simulink library "downlink_4c2t_lib"  (Simulink 8.7)
settings: Solver=ode45  StartTime=0.0  StopTime=10.0  RelTol=1e-3
PreLoadFcn:
  | LutContent = LUTS.ENTRIES;
InitFcn:
  | LutContent = LUTS.ENTRIES;
values from neighbouring files (symbols this model uses):
  cordic_gain = 1.8    [setup_downlink_4c2t.m]
undefined symbols (not defined in the file or in its folder): AdvDSPBDMemDisplay, dpoly, evalAionMaskParam, LUTS, UseDontCare, value
libraries: DSPBAPrim x42, DSPBAModelBus x10, DSPBAVectorUtil x2, downlink_4c2t_cordic_lib x1
settings Model: Creator=VMAUER  LastModifiedBy=5g

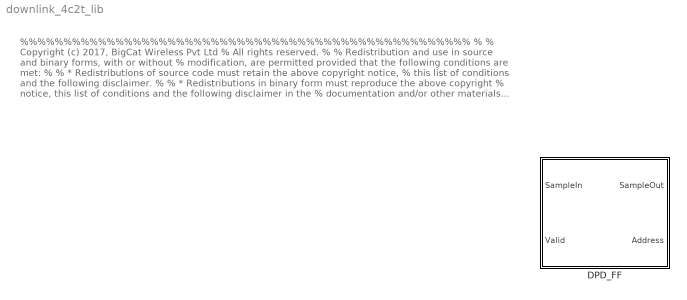
== system downlink_4c2t_lib ==
  note: %%%%%%%%%%%%%%%%%%%%%%%%%%%%%%%%%%%%%%%%%%%%%%%%%%%%
      |  %
      |  % Copyright (c) 2017, BigCat Wireless Pvt Ltd
      |  % All rights reserved.
      |  %
      |  % Redistribution and use in source and binary forms, with or without
      |  % modification, are permitted provided that the following conditions are met:
      |  %
      |  %     * Redistributions of source code must retain the above copyright notice,
      |  %       this list of conditions and the following disclaimer.
      |  %
      |  %     * Redistributions in binary form must reproduce the above copyright
      |  %       notice, this list of conditions and the following disclaimer in the
      |  %       documentation and/or other materials provided with the distribution.
      |  %
      |  %     * Neither the name of the copyright holder nor the names of its contributors
      |  %       may be used to endorse or promote products derived from this software
      |  %       without specific prior written permission.
      |  %
      |  %
      |  %
      |  % THIS SOFTWARE IS PROVIDED BY THE COPYRIGHT HOLDERS AND CONTRIBUTORS "AS IS"
      |  % AND ANY EXPRESS OR IMPLIED WARRANTIES, INCLUDING, BUT NOT LIMITED TO, THE
      |  % IMPLIED WARRANTIES OF MERCHANTABILITY AND FITNESS FOR A PARTICULAR PURPOSE ARE
      |  % DISCLAIMED. IN NO EVENT SHALL THE COPYRIGHT HOLDER OR CONTRIBUTORS BE LIABLE
      |  % FOR ANY DIRECT, INDIRECT, INCIDENTAL, SPECIAL, EXEMPLARY, OR CONSEQUENTIAL
      |  % DAMAGES (INCLUDING, BUT NOT LIMITED TO, PROCUREMENT OF SUBSTITUTE GOODS OR
      |  % SERVICES; LOSS OF USE, DATA, OR PROFITS; OR BUSINESS INTERRUPTION) HOWEVER
      |  % CAUSED AND ON ANY THEORY OF LIABILITY, WHETHER IN CONTRACT, STRICT LIABILITY,
      |  % OR TORT (INCLUDING NEGLIGENCE OR OTHERWISE) ARISING IN ANY WAY OUT OF THE USE
      |  % OF THIS SOFTWARE, EVEN IF ADVISED OF THE POSSIBILITY OF SUCH DAMAGE.
      |  %
      |   %%%%%%%%%%%%%%%%%%%%%%%%%%%%%%%%%%%%%%%%%%%%%%%%%%%%%
  DPD_FF : Subsystem  mask{LutContent=LUTS.ENTRIES, CoefWidth=16, Coeff_fractionwidth=11, DataWidth=16, fractionwidth=15, LutUpdateAddress=512, LutUpdateCoeff1=513, LutUpdateCoeff2=514, LutUpdateCoeff3=515, LutUpdateCoeff4=516, LutUpdateCoeff5=517, LutUpdateCoeff6=518, LutUpdateCoeff7=519, LutUpdateCoeff8=520, DPDReadBankAddress=521}
      mask prompts: LutContent "initial LUT content"; CoefWidth "Coefficient Width"; DataWidth "Data Width"; LutUpdateAddress "DPD LUT update address"; LutUpdateCoeff1 "DPD LUT update coeff 1"; LutUpdateCoeff2 "DPD LUT update coeff 2"; LutUpdateCoeff3 "DPD LUT update coeff 3"; LutUpdateCoeff4 "DPD LUT update coeff 4"; LutUpdateCoeff5 "DPD LUT update coeff 5"; LutUpdateCoeff6 "DPD LUT update coeff 6"; LutUpdateCoeff7 "DPD LUT update coeff 7"; LutUpdateCoeff8 "DPD LUT update coeff 8"; DPDReadBankAddress "DPD LUT read bank select"

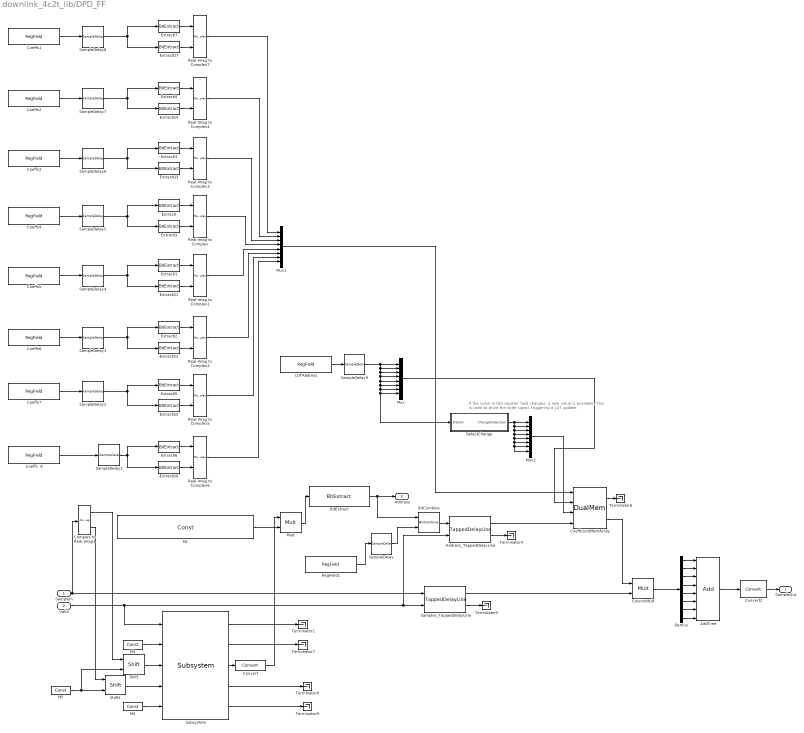
== system downlink_4c2t_lib/DPD_FF ==
  note: If the value in this register field changes, a new value is available.
      | This is used to drive the write signal, triggering a LUT update.
  SampleIn : Inport
  Valid : Inport  Port=2
  AddTree : DSPBAPrim/Add  primtype=add  nInputs=evalAionMaskParam(gcb,'value',1)  nOutputs=1  omode=Inherit via internal rule with word growth  otype=sfix(16)  scale=2^-15  rndmethod=Unbiased  factor=1  satmethod=Symmetric  shift_vec=[0 1 2 -1]  value=8  inPortNames=[' '; ' ';]  outPortNames=[' ']  dspbaimage=dspba_prim.jpg  text=fprintf('+');  style=Optimised  visibilities=1032+2^17+2^18+2^19  genFPC=off  floatRounding=correct  advOptions=[]  version=20130821
  Address_TappedDelayLine : DSPBAVectorUtil/TappedDelayLine  numTaps=size(LutContent, 2)  zeroOrOne=0  reverse=off
  BitCombine : DSPBAPrim/BitCombine  primtype=bitcombine  nInputs=2  nOutputs=1  omode=Inherit via internal rule  otype=sfix(16)  scale=2^-15  rndmethod=Unbiased  factor=1  satmethod=Symmetric  shift_vec=[0 1 2 -1]  value=0  inPortNames=['l'; 'h';]  outPortNames=[' ']  dspbaimage=dspba_prim.jpg  text=fprintf('[h,l]');  style=Optimised  visibilities=8+2  version=20090407
  BitExtract : DSPBAPrim/BitExtract  primtype=bitextract  nInputs=1  nOutputs=1  omode=Specify via dialog  otype=ufix(8)  scale=1  rndmethod=Unbiased  factor=1  satmethod=Symmetric  shift_vec=[0 1 2 -1]  value=log2(size(LutContent,1))  inPortNames=[' '; ' ';]  outPortNames=[' ']  dspbaimage=dspba_prim.jpg  text=fprintf('..%d', value);  style=Optimised  visibilities=8 + 1024  version=20090407
  CoefficientMemArray : DSPBAPrim/DualMem  primtype=dualmem  nInputs=4  nOutputs=2  omode=Specify via dialog  otype=sfix(CoefWidth)  scale=2^-Coeff_fractionwidth  rndmethod=Unbiased  factor=1  satmethod=Symmetric  shift_vec=[0 1 2 -1]  value=[LUTS.ENTRIES' LUTS.ENTRIES']'  inPortNames=['d'; 'a'; 'w'; 'a']  outPortNames=['q1'; 'q2']  dspbaimage=dspba_prim.jpg  text=fprintf('dmem%s',AdvDSPBDMemDisplay(UseDontCare));  style=Optimised  visibilities=8 + 1024 + 2^17  UseDontCare=on  TwinWritePorts=off  version=20141001
  Coeffs  8 : DSPBAModelBus/RegField  reg_name=LutUpdateCoeff8  reg_rwmode=Read/Write  reg_msb=2*DataWidth-1  reg_lsb=0  reg_mode=Specify via dialog  reg_type=ufix(2*DataWidth)  reg_scale=1  reg_init=0  reg_desc=I and Q coeffs for the next LUT entrance  reg_modal=off  reg_desc0=0  reg_desc1=0  reg_desc2=0  reg_desc3=0  reg_desc4=0  reg_desc5=0  reg_desc6=0  reg_desc7=0  reg_addr=520  SampleTime=-1  version=20090407
  Coeffs1 : DSPBAModelBus/RegField  reg_name=LutUpdateCoeff1  reg_rwmode=Read/Write  reg_msb=2*DataWidth-1  reg_lsb=0  reg_mode=Specify via dialog  reg_type=ufix(2*DataWidth)  reg_scale=1  reg_init=0  reg_desc=I and Q coeffs for the next LUT entrance  reg_modal=off  reg_desc0=0  reg_desc1=0  reg_desc2=0  reg_desc3=0  reg_desc4=0  reg_desc5=0  reg_desc6=0  reg_desc7=0  reg_addr=513  SampleTime=-1  version=20090407
  Coeffs2 : DSPBAModelBus/RegField  reg_name=LutUpdateCoeff2  reg_rwmode=Read/Write  reg_msb=2*DataWidth-1  reg_lsb=0  reg_mode=Specify via dialog  reg_type=ufix(2*DataWidth)  reg_scale=1  reg_init=0  reg_desc=I and Q coeffs for the next LUT entrance  reg_modal=off  reg_desc0=0  reg_desc1=0  reg_desc2=0  reg_desc3=0  reg_desc4=0  reg_desc5=0  reg_desc6=0  reg_desc7=0  reg_addr=514  SampleTime=-1  version=20090407
  Coeffs3 : DSPBAModelBus/RegField  reg_name=LutUpdateCoeff3  reg_rwmode=Read/Write  reg_msb=2*DataWidth-1  reg_lsb=0  reg_mode=Specify via dialog  reg_type=ufix(2*DataWidth)  reg_scale=1  reg_init=0  reg_desc=I and Q coeffs for the next LUT entrance  reg_modal=off  reg_desc0=0  reg_desc1=0  reg_desc2=0  reg_desc3=0  reg_desc4=0  reg_desc5=0  reg_desc6=0  reg_desc7=0  reg_addr=515  SampleTime=-1  version=20090407
  Coeffs4 : DSPBAModelBus/RegField  reg_name=LutUpdateCoeff4  reg_rwmode=Read/Write  reg_msb=2*DataWidth-1  reg_lsb=0  reg_mode=Specify via dialog  reg_type=ufix(2*DataWidth)  reg_scale=1  reg_init=0  reg_desc=I and Q coeffs for the next LUT entrance  reg_modal=off  reg_desc0=0  reg_desc1=0  reg_desc2=0  reg_desc3=0  reg_desc4=0  reg_desc5=0  reg_desc6=0  reg_desc7=0  reg_addr=516  SampleTime=-1  version=20090407
  Coeffs5 : DSPBAModelBus/RegField  reg_name=LutUpdateCoeff5  reg_rwmode=Read/Write  reg_msb=2*DataWidth-1  reg_lsb=0  reg_mode=Specify via dialog  reg_type=ufix(2*DataWidth)  reg_scale=1  reg_init=0  reg_desc=I and Q coeffs for the next LUT entrance  reg_modal=off  reg_desc0=0  reg_desc1=0  reg_desc2=0  reg_desc3=0  reg_desc4=0  reg_desc5=0  reg_desc6=0  reg_desc7=0  reg_addr=517  SampleTime=-1  version=20090407
  Coeffs6 : DSPBAModelBus/RegField  reg_name=LutUpdateCoeff6  reg_rwmode=Read/Write  reg_msb=2*DataWidth-1  reg_lsb=0  reg_mode=Specify via dialog  reg_type=ufix(2*DataWidth)  reg_scale=1  reg_init=0  reg_desc=I and Q coeffs for the next LUT entrance  reg_modal=off  reg_desc0=0  reg_desc1=0  reg_desc2=0  reg_desc3=0  reg_desc4=0  reg_desc5=0  reg_desc6=0  reg_desc7=0  reg_addr=518  SampleTime=-1  version=20090407
  Coeffs7 : DSPBAModelBus/RegField  reg_name=LutUpdateCoeff7  reg_rwmode=Read/Write  reg_msb=2*DataWidth-1  reg_lsb=0  reg_mode=Specify via dialog  reg_type=ufix(2*DataWidth)  reg_scale=1  reg_init=0  reg_desc=I and Q coeffs for the next LUT entrance  reg_modal=off  reg_desc0=0  reg_desc1=0  reg_desc2=0  reg_desc3=0  reg_desc4=0  reg_desc5=0  reg_desc6=0  reg_desc7=0  reg_addr=519  SampleTime=-1  version=20090407
  ColumnMult : DSPBAPrim/Mult  primtype=mult  nInputs=2  nOutputs=1  omode=Inherit via internal rule  otype=sfix(16)  scale=2^-11  rndmethod=Unbiased  factor=1  satmethod=Symmetric  shift_vec=[0 1 2 -1]  value=0  inPortNames=[' '; ' ';]  outPortNames=[' ']  dspbaimage=dspba_prim.jpg  text=fprintf('X');  style=Optimised  visibilities=8+2^18+2^19  floatPrecision=float32_m23  floatRounding=correct  advOptions=[]  version=20130115
  Complex to Real-Imag1 : ComplexToRealImag
  Convert : DSPBAPrim/Convert  primtype=convert  nInputs=1  nOutputs=1  omode=Specify via dialog  otype=ufix(10)  scale=2^-8  rndmethod=Truncate  factor=1  satmethod=None  shift_vec=[0 1 2 -1]  value=round([0:255]/17)  inPortNames=[' '; ' ';]  outPortNames=[' '; 'c']  dspbaimage=dspba_prim.jpg  text=fprintf('convert');  style=Optimised  visibilities=8+64+256+2^17  clipdetect=off  floatPrecision=float32_m23  advOptions=[]  version=20130211
  Convert2 : DSPBAPrim/Convert  primtype=convert  nInputs=1  nOutputs=1  omode=Specify via dialog  otype=sfix(DataWidth)  scale=2^-fractionwidth  rndmethod=Unbiased  factor=1  satmethod=None  shift_vec=[0 1 2 -1]  value=round([0:255]/17)  inPortNames=[' '; ' ';]  outPortNames=[' '; 'c']  dspbaimage=dspba_prim.jpg  text=fprintf('convert');  style=Optimised  visibilities=8+64+256  clipdetect=off  floatPrecision=float32_m23  advOptions=[]  version=20130211
  Demux : Demux  Outputs=8
  DetectChange : Subsystem
  ExtractI{,1..7} (8 alike) : DSPBAPrim/BitExtract  primtype=bitextract  nInputs=1  nOutputs=1  omode=Specify via dialog  otype=sfix(CoefWidth)  scale=2^-Coeff_fractionwidth  rndmethod=Unbiased  factor=1  satmethod=Symmetric  shift_vec=[0 1 2 -1]  value=CoefWidth  inPortNames=[' '; ' ';]  outPortNames=[' ']  dspbaimage=dspba_prim.jpg  text=fprintf('..%d', value);  style=Optimised  visibilities=8 + 1024  version=20090407
  ExtractQ{,1..3,5..6} (6 alike) : DSPBAPrim/BitExtract  primtype=bitextract  nInputs=1  nOutputs=1  omode=Specify via dialog  otype=sfix(CoefWidth)  scale=2^-Coeff_fractionwidth  rndmethod=Unbiased  factor=1  satmethod=Symmetric  shift_vec=[0 1 2 -1]  value=0  inPortNames=[' '; ' ';]  outPortNames=[' ']  dspbaimage=dspba_prim.jpg  text=fprintf('..%d', value);  style=Optimised  visibilities=8 + 1024  version=20090407
  ExtractQ4 : DSPBAPrim/BitExtract  primtype=bitextract  nInputs=1  nOutputs=1  omode=Specify via dialog  otype=sfix(DataWidth)  scale=2^-Coeff_fractionwidth  rndmethod=Unbiased  factor=1  satmethod=Symmetric  shift_vec=[0 1 2 -1]  value=0  inPortNames=[' '; ' ';]  outPortNames=[' ']  dspbaimage=dspba_prim.jpg  text=fprintf('..%d', value);  style=Optimised  visibilities=8 + 1024  version=20090407
  ExtractQ7 : DSPBAPrim/BitExtract  primtype=bitextract  nInputs=1  nOutputs=1  omode=Specify via dialog  otype=sfix(DataWidth)  scale=2^-Coeff_fractionwidth  rndmethod=Unbiased  factor=1  satmethod=Symmetric  shift_vec=[0 1 2 -1]  value=0  inPortNames=[' '; ' ';]  outPortNames=[' ']  dspbaimage=dspba_prim.jpg  text=fprintf('..%d', value);  style=Optimised  visibilities=8 + 1024  version=20090407
  LUTAddress : DSPBAModelBus/RegField  reg_name=LutUpdateAddress  reg_rwmode=Read/Write  reg_msb=ceil(log2(size(LutContent,1)))  reg_lsb=0  reg_mode=Specify via dialog  reg_type=ufix(log2(size(LutContent,1)) + 1)  reg_scale=1  reg_init=0  reg_desc=LUT address for Coeff update  reg_modal=off  reg_desc0=0  reg_desc1=0  reg_desc2=0  reg_desc3=0  reg_desc4=0  reg_desc5=0  reg_desc6=0  reg_desc7=0  reg_addr=512  SampleTime=-1  version=20090407
  M1 : DSPBAPrim/Const  primtype=const  nInputs=0  nOutputs=1  omode=Specify via dialog  otype=uint(8)  scale=1  rndmethod=Unbiased  factor=1  satmethod=Symmetric  shift_vec=[0 1 2 -1]  value=size(LutContent, 1) * (1/cordic_gain)  inPortNames=['+'; '+';]  outPortNames=[' ']  dspbaimage=dspba_prim.jpg  text=fprintf('%s', num2str(value));  style=Optimised  visibilities=8 + 1024  floatPrecision=float32_m23  version=20120820
  M3 : DSPBAPrim/Const  primtype=const  nInputs=0  nOutputs=1  omode=Specify via dialog  otype=sfix(16)  scale=2^-13  rndmethod=Unbiased  factor=1  satmethod=Symmetric  shift_vec=[0 1 2 -1]  value=0  inPortNames=['+'; '+';]  outPortNames=[' ']  dspbaimage=dspba_prim.jpg  text=fprintf('%s', num2str(value));  style=Optimised  visibilities=8 + 1024  floatPrecision=float32_m23  version=20120820
  M4 : DSPBAPrim/Const  primtype=const  nInputs=0  nOutputs=1  omode=Specify via dialog  otype=sfix(16)  scale=2^-15  rndmethod=Unbiased  factor=1  satmethod=Symmetric  shift_vec=[0 1 2 -1]  value=0  inPortNames=['+'; '+';]  outPortNames=[' ']  dspbaimage=dspba_prim.jpg  text=fprintf('%s', num2str(value));  style=Optimised  visibilities=8 + 1024  floatPrecision=float32_m23  version=20120820
  M5 : DSPBAPrim/Const  primtype=const  nInputs=0  nOutputs=1  omode=Specify via dialog  otype=uint(4)  scale=2^0  rndmethod=Unbiased  factor=1  satmethod=Symmetric  shift_vec=[0 1 2 -1]  value=2  inPortNames=['+'; '+';]  outPortNames=[' ']  dspbaimage=dspba_prim.jpg  text=fprintf('%s', num2str(value));  style=Optimised  visibilities=8 + 1024  floatPrecision=float32_m23  version=20120820
  Mult : DSPBAPrim/Mult  primtype=mult  nInputs=2  nOutputs=1  omode=Inherit via internal rule  otype=double  scale=1  rndmethod=Unbiased  factor=1  satmethod=Symmetric  shift_vec=[0 1 2 -1]  value=0  inPortNames=[' '; ' ';]  outPortNames=[' ']  dspbaimage=dspba_prim.jpg  text=fprintf('X');  style=Optimised  visibilities=8  floatPrecision=float32_m23  floatRounding=correct  advOptions=[]  version=20130115
  Mux : Mux  Inputs=8
  Mux1 : Mux  Inputs=8
  Mux2 : Mux  Inputs=8
  Real-Imag to Complex{,1..7} (8 alike) : RealImagToComplex
  RegField1 : DSPBAModelBus/RegField  reg_name=DPDReadBankAddress  reg_rwmode=Read/Write  reg_msb=0  reg_lsb=0  reg_mode=Specify via dialog  reg_type=ufix(1)  reg_scale=1  reg_init=0  reg_desc=Selects LUT bank  reg_modal=off  reg_desc0=0  reg_desc1=0  reg_desc2=0  reg_desc3=0  reg_desc4=0  reg_desc5=0  reg_desc6=0  reg_desc7=0  reg_addr=521  SampleTime=-1  version=20090407
  SampleDelay{,1..9} (10 alike) : DSPBAPrim/SampleDelay  primtype=sampdelay  nInputs=1  nOutputs=1  omode=Inherit via internal rule  otype=sfix(16)  scale=2^-15  rndmethod=Unbiased  factor=1  satmethod=Symmetric  shift_vec=[0 1 2 -1]  value=1  inPortNames=[' '; ' ';]  outPortNames=[' ']  dspbaimage=dspba_prim.jpg  text=dpoly(1, eye(1,value+1), 'z')  style=Optimised  visibilities=8 + 1024 + 2^17 + 2^18  flexible=off  slackgroup=0  augmented=0  version=20090407  advOptions=[]
  Samples_TappedDelayLine : DSPBAVectorUtil/TappedDelayLine  numTaps=size(LutContent, 2)  zeroOrOne=0  reverse=off
  Shift : DSPBAPrim/Shift  primtype=shift  nInputs=2  nOutputs=1  omode=Specify via dialog  otype=sfix(16)  scale=2^-15  rndmethod=Unbiased  factor=1  satmethod=Symmetric  shift_vec=[0 1 2 -1]  value=0  inPortNames=['a'; 'b';]  outPortNames=[' ']  dspbaimage=dspba_prim.jpg  text=fprintf('a >> b');  style=Optimised  visibilities=8  version=20090407
  Shift1 : DSPBAPrim/Shift  primtype=shift  nInputs=2  nOutputs=1  omode=Specify via dialog  otype=sfix(16)  scale=2^-15  rndmethod=Unbiased  factor=1  satmethod=Symmetric  shift_vec=[0 1 2 -1]  value=0  inPortNames=['a'; 'b';]  outPortNames=[' ']  dspbaimage=dspba_prim.jpg  text=fprintf('a >> b');  style=Optimised  visibilities=8  version=20090407
  Subsystem : downlink_4c2t_cordic_lib/Subsystem  stages=dpd_stages  angle_bits=dpd_xy_angle_bits  angle_frac_bits=dpd_xy_angle_fract_bits  xy_bits=dpd_xy_bits  xy_frac_bits=dpd_xy_fract_bits
  Terminator{1,4..9} (7 alike) : Terminator
  SampleOut : Outport
  Address : Outport  Port=2
  wires:
  Coeffs4/1 -> SampleDelay5/1
  Complex to Real-Imag1/1 -> Shift/1
  Complex to Real-Imag1/2 -> Shift1/1
  CoefficientMemArray/2 -> ColumnMult/1
  AddTree/1 -> Convert2/1
  Address_TappedDelayLine/2 -> Terminator4/1
  Samples_TappedDelayLine/2 -> Terminator5/1
  Samples_TappedDelayLine/1 -> ColumnMult/2
  BitCombine/1 -> Address_TappedDelayLine/1
  Address_TappedDelayLine/1 -> CoefficientMemArray/4
  CoefficientMemArray/1 -> Terminator6/1
  Convert2/1 -> SampleOut/1
  ExtractI/1 -> Real-Imag to Complex/1
  ExtractQ/1 -> Real-Imag to Complex/2
  RegField1/1 -> SampleDelay/1
  SampleIn/1 -> Samples_TappedDelayLine/1, Complex to Real-Imag1/1
  Valid/1 -> Subsystem/1, Address_TappedDelayLine/2, Samples_TappedDelayLine/2
  M1/1 -> Mult/2
  BitExtract/1 -> Address/1, BitCombine/1
  LUTAddress/1 -> SampleDelay9/1
  Mux/1 -> CoefficientMemArray/2
  Coeffs5/1 -> SampleDelay4/1
  ExtractI1/1 -> Real-Imag to Complex1/1
  ExtractQ1/1 -> Real-Imag to Complex1/2
  Coeffs6/1 -> SampleDelay3/1
  ExtractI2/1 -> Real-Imag to Complex2/1
  ExtractQ2/1 -> Real-Imag to Complex2/2
  Coeffs3/1 -> SampleDelay6/1
  ExtractI3/1 -> Real-Imag to Complex3/1
  ExtractQ3/1 -> Real-Imag to Complex3/2
  Coeffs2/1 -> SampleDelay7/1
  ExtractI4/1 -> Real-Imag to Complex4/1
  ExtractQ4/1 -> Real-Imag to Complex4/2
  Coeffs7/1 -> SampleDelay2/1
  ExtractI5/1 -> Real-Imag to Complex5/1
  ExtractQ5/1 -> Real-Imag to Complex5/2
  Coeffs  8/1 -> SampleDelay1/1
  ExtractI6/1 -> Real-Imag to Complex6/1
  ExtractQ6/1 -> Real-Imag to Complex6/2
  Coeffs1/1 -> SampleDelay8/1
  ExtractI7/1 -> Real-Imag to Complex7/1
  ExtractQ7/1 -> Real-Imag to Complex7/2
  Real-Imag to Complex/1 -> Mux1/4
  Real-Imag to Complex1/1 -> Mux1/5
  Real-Imag to Complex2/1 -> Mux1/6
  Real-Imag to Complex5/1 -> Mux1/7
  Real-Imag to Complex6/1 -> Mux1/8
  Real-Imag to Complex3/1 -> Mux1/3
  Real-Imag to Complex4/1 -> Mux1/2
  Real-Imag to Complex7/1 -> Mux1/1
  Mux1/1 -> CoefficientMemArray/1
  DetectChange/1(ChangeDetected) -> Mux2/2, Mux2/3, Mux2/4, Mux2/5, Mux2/6, Mux2/7, Mux2/8, Mux2/1
  Mux2/1 -> CoefficientMemArray/3
  ColumnMult/1 -> Demux/1
  Demux/1 -> AddTree/1
  Demux/2 -> AddTree/2
  Demux/3 -> AddTree/3
  Demux/4 -> AddTree/4
  Demux/5 -> AddTree/5
  Demux/6 -> AddTree/6
  Demux/7 -> AddTree/7
  Demux/8 -> AddTree/8
  M3/1 -> Subsystem/2
  M4/1 -> Subsystem/5
  Subsystem/1 -> Terminator1/1
  Subsystem/2 -> Terminator7/1
  Subsystem/4 -> Terminator8/1
  Subsystem/5 -> Terminator9/1
  Mult/1 -> BitExtract/1
  Subsystem/3 -> Convert/1
  Convert/1 -> Mult/1
  SampleDelay/1 -> BitCombine/2
  SampleDelay1/1 -> ExtractQ6/1, ExtractI6/1
  SampleDelay2/1 -> ExtractQ5/1, ExtractI5/1
  SampleDelay3/1 -> ExtractI2/1, ExtractQ2/1
  SampleDelay4/1 -> ExtractI1/1, ExtractQ1/1
  SampleDelay5/1 -> ExtractI/1, ExtractQ/1
  SampleDelay6/1 -> ExtractI3/1, ExtractQ3/1
  SampleDelay7/1 -> ExtractI4/1, ExtractQ4/1
  SampleDelay8/1 -> ExtractI7/1, ExtractQ7/1
  SampleDelay9/1 -> Mux/4, Mux/5, Mux/6, Mux/7, Mux/8, DetectChange/1(DataIn), Mux/3, Mux/2, Mux/1
  Shift/1 -> Subsystem/3
  Shift1/1 -> Subsystem/4
  M5/1 -> Shift/2, Shift1/2

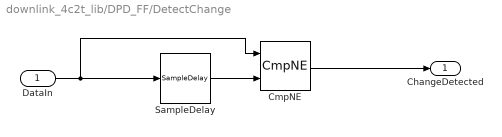
== system downlink_4c2t_lib/DPD_FF/DetectChange ==
  DataIn : Inport
  CmpNE : DSPBAPrim/CmpNE  primtype=cmpne  nInputs=2  nOutputs=1  omode=boolean  otype=sfix(16)  scale=2^-15  rndmethod=Unbiased  factor=1  satmethod=Symmetric  shift_vec=[0 1 2 -1]  value=0  inPortNames=[' '; ' ';]  outPortNames=[' ']  dspbaimage=dspba_prim.jpg  text=fprintf('~=');  style=Optimised  visibilities=0  advOptions=[]  version=20130117
  SampleDelay : DSPBAPrim/SampleDelay  primtype=sampdelay  nInputs=1  nOutputs=1  omode=Inherit via internal rule  otype=sfix(16)  scale=2^-15  rndmethod=Unbiased  factor=1  satmethod=Symmetric  shift_vec=[0 1 2 -1]  value=1  inPortNames=[' '; ' ';]  outPortNames=[' ']  dspbaimage=dspba_prim.jpg  text=dpoly(1, eye(1,value+1), 'z')  style=Optimised  visibilities=8 + 1024 + 2^17 + 2^18  flexible=off  slackgroup=0  augmented=0  version=20090407  advOptions=[]
  ChangeDetected : Outport
  wires:
  CmpNE/1 -> ChangeDetected/1
  DataIn/1 -> CmpNE/1, SampleDelay/1
  SampleDelay/1 -> CmpNE/2
